simulink library "ScienceStim2_Lib"  (Simulink 8.0)
settings: Solver=ode45  SolverMode=SingleTasking  StartTime=0.0  StopTime=10.0  RelTol=1e-3
settings Model: Creator=henrik  LastModifiedBy=Thomas Schauer

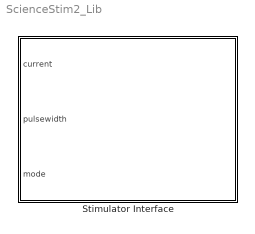
== system ScienceStim2_Lib ==
  Stimulator Interface : Subsystem  mask(Stimulator Interface (RehaStim2 - Hasomed GmbH)){sampletime=0.05, comport=sciencemode2, stim_channels=[1 2 5 6], maintime=0, grouptime=8, lf_channels=[], lf_factor=[], dtflag=on}
      mask prompts: sampletime "Sample Time in ms:"; comport "Serial Port:"; stim_channels "Channels to be Stimulated:"; maintime "Main Pulse Interval in ms (only in steps of 0.5 ms):"; grouptime "Inter Pulse Interval in ms (only in steps of 0.5 ms, > 8ms):"; lf_channels "Low Frequency Channels:"; lf_factor "Low Frequency Factor:"; dtflag "Enable doublets and triplets"
      mask help: Communication to the 8-channel RehaStim2 Stimulator (HASOMED GmbH)
      mask init:
      | load_system simulink
      | %---------------------------------------------------------------------------
      | % Mute Output
      | % % Get the mask parameter values. This is a cell array of strings.
      | % maskStr = get_param(gcb, 'MaskValues');
      | % % The outflag is the 8th mask parameter.
      | %     block = 'mute period [ms]';
      | %     system_block = [gcb '/' block];
      | %     srcblock = 'S-Function';
      | %     system_srcblock = [gcb '/' srcblock];
      | %     pos = get_param(system_block, 'position');
      | %     blocktype = get_param(system_block, 'blocktype');
      | % % Check the value selected 
      | % if strcmp(maskStr{8}, 'on'),
      | %     if ~strcmp(blocktype, 'Outport')
      | %         delete_line(gcb, [srcblock '/1'], [block '/1']);
      | %         delete_block(system_block);
      | %         add_block('simulink/Sinks/Out1', system_block, 'position', pos);
      | %         add_line(gcb, [srcblock '/1'], [block '/1']);
      | %     end
      | % else
      | %     if ~strcmp(blocktype, 'Terminator')
      | %         delete_line(gcb, [srcblock '/1'], [block '/1']);
      | %         delete_block(system_block);
      | %         add_block('simulink/Sinks/Terminator', system_block, 'position', pos);
      | %         add_line(gcb, [srcblock '/1'], [block '/1']);
      | %     end
      | % end
      | %---------------------------------------------------------------------------
      | % Mode input
      | % Get the mask parameter values. This is a cell array of strings.
      | maskStr = get_param(gcb, 'MaskValues');
      | % The doublet / triplet flag is the 9th mask parameter.
      |     block = 'mode';
      |     system_block = [gcb '/' block];
      |     sinkblock = 'S-Function';
      |     system_sinkblock = [gcb '/' sinkblock];
      |     pos = get_param(system_block, 'position');
      |     blocktype = get_param(system_block, 'blocktype');
      | % Check the value selected 
      | if strcmp(maskStr{8}, 'on'),
      |     if ~strcmp(blocktype, 'Inport')
      |         delete_line(gcb, [block '/1'], [sinkblock '/3']);
      |         delete_block(system_block);
      |         add_block('simulink/Sources/In1', system_block, 'Port', '3', 'position', pos);
      |         add_line(gcb, [block '/1'], [sinkblock '/3']);
      |     end
      | else % disable mode input, setit to zeros
      |     if ~strcmp(blocktype, 'Constant')
      |         delete_line(gcb, [block '/1'], [sinkblock '/3']);
      |         delete_block(system_block);
      |         add_block('simulink/Sources/Constant', system_block, 'position', pos);
      |         set_param(system_block, 'value', 'zeros(1, length(stim_channels))');
      |         add_line(gcb, [block '/1'], [sinkblock '/3']);
      |     end
      |     % Make sure Group time is large enough if doublet / triplet is off
      |     % It must be at least 1.5 x Number_of_Channels, so we add 0.5 to that
      |     grouptime = 1.5 * length(stim_channels) + 0.5;
      | end
      | 
      | 
      | %---------------------------------------------------------------------------
      | % default minimal Mask Display string
      | MDstr=['image(imread(''RehaStim-background.png''), [0.05 0.25 0.9 0.9]);'...
      |     'port_label(''input'', 1, ''current'');'...
      |     'port_label(''input'', 2, ''pulsewidth'');'...
      |     'text(0.25,0.1,[''Serial Port Index: '' num2str(comport)],''horizontalAlignment'',''left'',''verticalAlignment'',''bottom'');'...
      |     'text(0.25,0,[''Channels: '' num2str(stim_channels)],''horizontalAlignment'',''left'',''verticalAlignment'',''bottom'');'];
      | % get the number of inputs and outputs and add additional labels if needed
      | num_ports = get_param(gcb, 'Ports');
      | num_inputs = num_ports(1);
      | num_outputs = num_ports(2);
      | if num_inputs >= 3
      |     MDstr = [MDstr 'port_label(''input'', 3, ''mode'');'];
      | end
      | if num_outputs >= 1
      |     MDstr = [MDstr 'port_label(''output'', 1, ''mute time [ms]'');'];
      | end
      | set_param(gcb, 'MaskDisplay', MDstr)
      mask Help: eval('open(''ScienceStim2_Help.html'')')
      mask TypeOptions comport: sciencemode2 | ttyUSB0 | ttyUSB1 | ttyUSB2 | ttyUSB3 | COM1 | COM2 | COM3 | COM4 | COM5 | COM6 | COM6 | COM7 | COM8
      mask Callback dtflag:
      | % Get the mask parameter values. This is a cell array of strings.
      | maskStr = get_param(gcb,'MaskValues');
      | % The doublet / triplet flag is the 9th mask parameter.
      | % Check the value selected
      | if strcmp(maskStr{8},'on'),
      |     % show associated parameter (Group Time)
      |     set_param(gcb,'MaskVisibilities',{'on';'on';'on';'on';'on';'on';'on';'on'})
      | else
      |     % hide associated parameter (Group Time)
      |     set_param(gcb,'MaskVisibilities',{'on';'on';'on';'on';'off';'on';'on';'on'})
      | end
      mask Display: image(imread('RehaStim-background.png'), [0.05 0.25 0.9 0.9]);port_label('input', 1, 'current');port_label('input', 2, 'pulsewidth');text(0.25,0.1,['Serial Port Index: ' num2str(comport)],'horizontalAlignment','left','verticalAlignment','bottom');text(0.25,0,['Channels: ' num2str(stim_channels)],'horizontalAlignment','left','verticalAlignment','bottom');port_label('input', 3, 'mode');

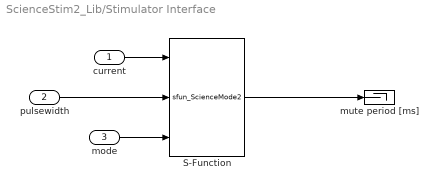
== system ScienceStim2_Lib/Stimulator Interface ==
  current : Inport
  pulsewidth : Inport  Port=2
  mode : Inport  Port=3
  S-Function : S-Function  FunctionName=sfun_ScienceMode2  Parameters=sampletime,comport,stim_channels,maintime,grouptime,0,lf_channels,lf_factor  EnableBusSupport=off
  mute period [ms] : Terminator
  wires:
  current/1 -> S-Function/1
  pulsewidth/1 -> S-Function/2
  S-Function/1 -> mute period [ms]/1
  mode/1 -> S-Function/3
